simulink model "NDI"  (R2022a)
settings: Solver=ode4  StartTime=0  StopTime=100  FixedStep=fcs.Ts  RelTol=1e-3
undefined symbols (not defined in the file or in its folder): Aactuator, ac, AeroCoeff, ControlAllocation, DUmax, DUmin, EngineTable, F, fcs, ft, g, hground, IC, kg, LandingGear, Light, m, MIL, Mode_deflection_aileron, Mode_deflection_elevator, Mode_deflection_rudder, Mode_deflection_TVC_y, Mode_deflection_TVC_z, N, Ninv_2nozzle, Ninv_no_nozzle, PIController, s, Sensor, sigbuilder_block, slug, state0, sysID_DAQ, sysID_OBES, Umax_2nozzle, Umax_no_nozzle, Umin_2nozzle, Umin_no_nozzle, WMM2020
libraries: aerolibconvert2 x31, slpidlib x11, simulink x6, sharedutil x4, aerolibatmos2 x3, aerolibwind2 x3, aerolibbdyn x3, aerolibgravity2 x2, sharedtransform x1
(part 1 of 13)
settings Model: Creator=User
settings SolverCC: AlgebraicLoopSolver=TrustRegion
settings DataIOCC: FinalStateName=xFinalOP  InitialState=xFinalOP  SaveOperatingPoint=on  ReturnWorkspaceOutputs=off
settings DebuggingCC: UnconnectedInputMsg=warning  UnconnectedOutputMsg=warning  UnconnectedLineMsg=warning  SFMachineParentedDataDiag=warning
settings ConfigComp: DVTestSuiteOptimization=Auto  DVDetectOutOfBounds=on

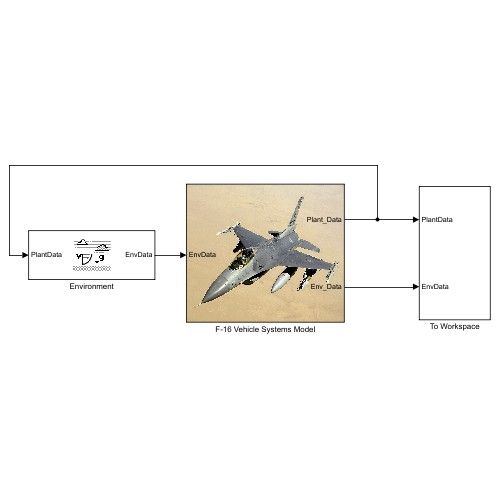
[thumbnail: Simulink's stored preview of the top-level diagram]
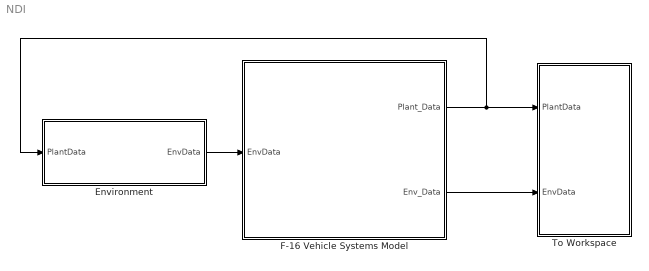
== system NDI ==
  Environment : Subsystem
      mask Display:
      | image('aeroenvironment.bmp','center')
      | % 左側 "Icon transparency" 欄位已選擇 "Opaque with ports"，所以埠名稱會自動顯示，不用再宣告
      | % port_label('input',1,'PlantData')
      | % port_label('output',1,'EnvData')
  F-16 Vehicle Systems Model : Subsystem
      mask Display:
      | proj = currentProject;   % 返回一個專案物件proj 代表當前打開的Project專案
      | filepath = fullfile(proj.RootFolder,'\image\F-16_wikipedia.jpg');
      | image(filepath,'center');
      | % 左側 "Icon transparency" 欄位已選擇 "Opaque with ports"，所以埠名稱會自動顯示，不用再宣告
      | % port_label('input',1,'EnvData')
      | % port_label('output',1,'Plant_Data')
      | % port_label('output',2,'Env_Data')
  To Workspace : Subsystem
  wires:
  F-16 Vehicle Systems Model/1(Plant_Data) -> Environment/1(PlantData), To Workspace/1(PlantData)
  F-16 Vehicle Systems Model/2(Env_Data) -> To Workspace/2(EnvData)
  Environment/1(EnvData) -> F-16 Vehicle Systems Model/1(EnvData)

== system NDI/Environment ==
  note: p, q, r
  note: u, v, w
  note: Wind Models
  note: Atmosphere Model
  note: Altitude must be less than 20000 m (approximately 65620 feet).
  note: 建模注意： EnvData Bus 內要指定公制/英制單位
  note: Magnetic Field
  note: Gravity Model
  note: TODO: 改用這個現成模塊...
      | 但NDI控制器內的重力g是用常數，將產生誤差...
  note: TODO: 改用這個現成模塊...
      | 參考MATLAB Help範例 Quadcopter Project
  note: TODO: 改用現成模塊，改成英制。
      | NDI控制器，不會產生誤差，因為可轉成C程式碼
  note: TODO: 參考MATLAB Help範例 HL-20
      | 將風速效應加到氣動力攻角、側滑角、qbar、Mach、V
  In Bus Element1 : Inport  PortName=PlantData  Element=altitude
  In Bus Element2 : Inport  PortName=PlantData  Element=altitude
  In Bus Element3 : Inport  PortName=PlantData  Element=Vt
  In Bus Element4 : Inport  PortName=PlantData  Element=Vt
  In Bus Element5 : Inport  PortName=PlantData  Element=Vt
  In Bus Element : Inport  PortName=PlantData  Element=DCM_be
  COESA Atmosphere Model : aerolibatmos2/COESA Atmosphere Model  Commented=on  units=English (Velocity in ft/s)  spec=1976 COESA-extended U.S. Standard Atmosphere  model=Profile  profile_var=High temperature  profile_percent=1%  profile_alt=5 km (16404 ft)  envelope_var=High temperature  envelope_percent=1%  action=Warning
  Density Conversion : aerolibconvert2/Density Conversion  IU=kg/m^3  OU=slug/ft^3
      settings: SourceProductBaseCode=AE
  Discrete Wind Gust Model : aerolibwind2/Discrete Wind Gust Model  Commented=on  units=English (Velocity in ft/s)  Gx=on  Gy=on  Gz=on  t_0=5  d_m=[120 120 80]  v_m=[3.5 3.5 3.0]
  Dryden Wind Turbulence Model (Continuous (+q +r)) : aerolibwind2/Dryden Wind Turbulence Model  (Continuous (+q -r))  Commented=on  units=English (Velocity in ft/s)  spec=MIL-F-8785C  model=Continuous Dryden (+q +r)  W20=15  Wdeg=0  TurbProb=10^-2 - Light  L_high=533.4  Wingspan=10  ts=0.1  Seed=[23341 23342 23343 23344]  T_on=on
  Dynamic Pressure : Subsystem
  Geoid Height : aerolibgravity2/Geoid Height  Commented=on  units=English  gtype=EGM96  datafile='geoidegm96grid'  dtype=double  action=Warning
      settings: AttributesFormatString=EGM2008 Geoid Data Unavailable  SourceProductBaseCode=AE
  ISA Atmosphere Model : aerolibatmos2/ISA Atmosphere Model  Commented=on  custom=off  g=9.80665  gamma=1.4  R=287.0531  L=0.0065  h_trop=11000  h_strat=20000  rho0=1.225  P0=101325  T0=288.15  h0=0
  "ISP " : Subsystem
  Length Conversion : aerolibconvert2/Length Conversion  IU=ft  OU=m
  Mach Number : Subsystem
  Magnetic Field : Constant  Value=[0 0 0]
  Manual Switch : ManualSwitch
  Manual Switch1 : ManualSwitch  CurrentSetting=0
  Pressure Altitude : aerolibatmos2/Pressure Altitude  Commented=on  units=English  action=Warning
      settings: SourceProductBaseCode=AE
  Sum : Sum  Commented=on  Inputs=+++
  Velocity Conversion : aerolibconvert2/Velocity Conversion  IU=m/s  OU=ft/s
  "WGS84 Gravity Model  " : GravityWGS84  Commented=on  units=English
  Wind Shear Model : aerolibwind2/Wind Shear Model  Commented=on  units=English (Velocity in ft/s)  phase=Category C - Terminal Flight Phase  W_20=15  Wdeg=0
  World Magnetic Model : aerolibgravity2/World Magnetic Model  Commented=on  model=WMM2020 (2020-2025)  customFile='WMM2020.COF'  units=English  time_in=on  month=January  day=1  year=2020  action=Error  h_out=off  dec_out=off  inc_out=off  ti_out=off
      settings: SourceProductBaseCode=AE
  gravity (ft/s^2) : Constant  Value=g
  hground (ft) : Constant  Value=hground
  no wind : Constant  Value=[0 0 0]
  no wind1 : Constant  Value=[0 0 0]
  r2d1 : Gain  Commented=on  Gain=-1  SaturateOnIntegerOverflow=on  OutDataTypeStr=Inherit: Same as input  ParamDataTypeStr=Inherit: Same as input
  r2d2 : Gain  Gain=-1  SaturateOnIntegerOverflow=on  OutDataTypeStr=Inherit: Same as input  ParamDataTypeStr=Inherit: Same as input
  Out Bus Element : Outport  PortName=EnvData  Element=Pressure
  Out Bus Element1 : Outport  PortName=EnvData  Element=AirDensity
  Out Bus Element2 : Outport  PortName=EnvData  Element=qbar
  Out Bus Element3 : Outport  PortName=EnvData  Element=Mach
  Out Bus Element4 : Outport  PortName=EnvData  Element=g
  Out Bus Element5 : Outport  PortName=EnvData  Element=hground
  Out Bus Element6 : Outport  PortName=EnvData  Element=MagneticField_NED
  Out Bus Element7 : Outport  PortName=EnvData  Element=AirTemperature_K
  Out Bus Element8 : Outport  PortName=EnvData  Element=SoundSpeed_ms
  Out Bus Element9 : Outport  PortName=EnvData  Element=WindVelocity
  Out Bus Element10 : Outport  PortName=EnvData  Element=WindAngularRates
  wires:
  "ISP "/1(T (K)) -> Out Bus Element7/1
  "ISP "/3(P (HPa)) -> Out Bus Element/1
  "ISP "/4(rho (kg/m^3)) -> Density Conversion/1, Out Bus Element1/1
  hground (ft)/1 -> Out Bus Element5/1
  gravity (ft/s^2)/1 -> Out Bus Element4/1  "Gravity_NED"
  Magnetic Field/1 -> Out Bus Element6/1  "MagneticField_NED"
  In Bus Element1/1 -> r2d2/1
  r2d2/1 -> Length Conversion/1  "h(ft)"
  Length Conversion/1 -> "ISP "/1(h(m))
  "ISP "/2(a (m/s)) -> Out Bus Element8/1, Velocity Conversion/1
  Mach Number/1(Mach) -> Out Bus Element3/1
  Dynamic Pressure/1(qbar) -> Out Bus Element2/1
  Density Conversion/1 -> Dynamic Pressure/2(rho)
  In Bus Element3/1 -> Dynamic Pressure/1(Vt)  "Vt (ft/s)"
  In Bus Element4/1 -> Mach Number/1(Vt)  "Vt (ft/s)"
  Velocity Conversion/1 -> Mach Number/2(a)
  COESA Atmosphere Model/3 -> Pressure Altitude/1
  r2d1/1 -> Dryden Wind Turbulence Model (Continuous (+q +r))/1, Wind Shear Model/1  "h(ft)"
  In Bus Element2/1 -> r2d1/1
  In Bus Element5/1 -> Discrete Wind Gust Model/1, Dryden Wind Turbulence Model (Continuous (+q +r))/2  "Vt (ft/s)"
  In Bus Element/1 -> Wind Shear Model/2, Dryden Wind Turbulence Model (Continuous (+q +r))/3
  Dryden Wind Turbulence Model (Continuous (+q +r))/1 -> Sum/2
  Discrete Wind Gust Model/1 -> Sum/3
  Wind Shear Model/1 -> Sum/1
  Dryden Wind Turbulence Model (Continuous (+q +r))/2 -> Manual Switch1/1  "WindAngularRates"
  Sum/1 -> Manual Switch/2  "WindVelocity"
  Manual Switch/1 -> Out Bus Element9/1
  no wind/1 -> Manual Switch/1
  Manual Switch1/1 -> Out Bus Element10/1
  no wind1/1 -> Manual Switch1/2
